simulink model "full_bridge_ac_dc_conv"  (R2019b)
settings: Solver=VariableStepAuto  StartTime=0.0  StopTime=0.2  RelTol=1e-3
libraries: powerlib x12, powerlib_extras x1
settings Model: Creator=SPS VISION  LastModifiedBy=SPS VISION

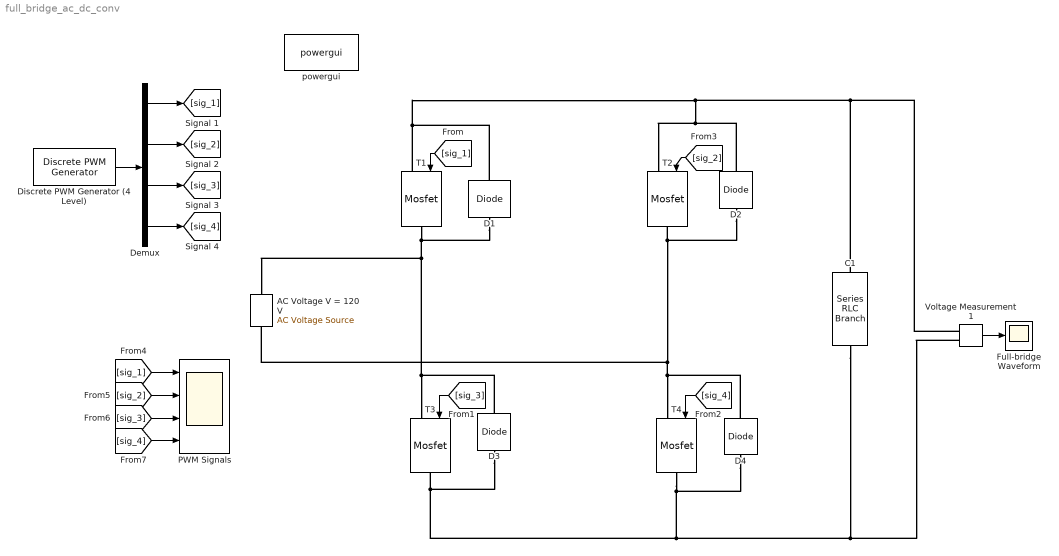
== system full_bridge_ac_dc_conv ==
  AC Voltage V = 120 V : powerlib/Electrical Sources/AC Voltage Source  Amplitude=120  Phase=0  Frequency=60  SampleTime=0  Measurements=None  BusType=swing  Pref=10e3  Qref=0  Qmin=-inf  Qmax=+inf
      settings: SourceProductName=Simscape Electrical
  C1 : powerlib/Elements/Series RLC Branch  LConnTagsString=__new0  RConnTagsString=__new0  BranchType=C  Resistance=1  Inductance=5e-3  SetiL0=off  InitialCurrent=0  Capacitance=1e-6  Setx0=off  InitialVoltage=0  Measurements=None
      settings: SourceProductName=Simscape Electrical
  D{1..4} (4 alike) : powerlib/Power Electronics/Diode  Ron=0.001  Lon=0  Vf=0.8  IC=0  UseSnubber=off  Rs=500  Cs=250e-9  Measurements=off
      settings: SourceProductName=Simscape Electrical
  Demux : Demux
  Discrete PWM Generator (4 Level) : powerlib_extras/Discrete  Control Blocks/Discrete PWM Generator  GeneratorMode="2-arm  bridge (4 pulses)"  Fc=600  Ts=5e-6  Internal=on  mIndex=0.4  Freq=60  Phase=0
      settings: SourceProductName=Simscape Electrical  SourceProductBaseCode=PS
  Full-bridge Waveform : Scope
  PWM Signals : Scope  NumInputPorts=4
  T{1..4} (4 alike) : powerlib/Power Electronics/Mosfet  Ron=0.1  Lon=0  Rd=0.01  Vfd=0  IC=0  Rs=1e5  Cs=inf  Measurements=off
      settings: SourceProductName=Simscape Electrical
  Voltage Measurement1 : powerlib/Measurements/Voltage Measurement  PhasorSimulation=off  OutputType=Complex  PSBequivalent=0
      settings: SourceProductName=Simscape Electrical
  powergui : powerlib/powergui  Priority=1  SimulationMode=Continuous  SampleTime=50e-6  frequency=60  Iterations=50  frequencyindice=60  Pbase=100e6  ErrMax=1e-4  UnitsV=kV  UnitsW=MW  buscounter=0  FunctionMessages=off  echomessages=off  EnableUseOfTLC=off  CurrentSourceSwitches=off  DisableSnubberDevices=off  DisableRonSwitches=off  DisableVfSwitches=off  DisplayEquations=off  AutomaticDiscreteSolvers=off  SolverType=Tustin/Backward Euler (TBE)  Interpol=off  ExternalGateDelay=off  methode=off  Ts=100  x0status=blocks  SPID=on  SwTol=0  HookPort=off  NonlinearTolerance=1e-4  nMaxIteration=100  ContinueOnMaxIteration=off  RestoreLinks=warning  ResistiveCurrentMeasurement=off  Frange=[0:2:500]  Ylog=off  Xlog=on  ShowGrid=off  save=off  variable=ZData  structure=0  ZoomFFT=off  StartTime=0.0  cycles=1  DisplayStyle=1  fundamental=60  FreqAxis=off  MaxFrequency=1000  frequencyindicesteady=1  RmsSteady=1  display=off
      settings: SourceProductName=Simscape Electrical
  wires:
  Discrete PWM Generator (4 Level)/1 -> Demux/1
  Demux/1 -> [sig_1]
  [sig_1] -> T1/1
  Demux/2 -> [sig_2]
  [sig_3] -> T3/1
  Voltage Measurement1/1 -> Full-bridge Waveform/1
  [sig_4] -> T4/1
  [sig_2] -> T2/1
  Demux/3 -> [sig_3]
  Demux/4 -> [sig_4]
  [sig_2] -> PWM Signals/2
  [sig_1] -> PWM Signals/1
  [sig_3] -> PWM Signals/3
  [sig_4] -> PWM Signals/4
  connections:
  C1/RConn1 -- Voltage Measurement1/LConn2 -- T4/RConn1 -- D4/LConn1 -- T3/RConn1 -- D3/LConn1
  D4/RConn1 -- T4/LConn1 -- D2/LConn1 -- T2/RConn1 -- AC Voltage V = 120 V/LConn1
  D3/RConn1 -- T3/LConn1 -- AC Voltage V = 120 V/RConn1 -- D1/LConn1 -- T1/RConn1
  C1/LConn1 -- Voltage Measurement1/LConn1 -- T2/LConn1 -- D2/RConn1 -- T1/LConn1 -- D1/RConn1
